simulink subsystem "State_Estimator"  (R2025b)
settings: Solver=VariableStepAuto  StartTime=0.0  StopTime=10.0  RelTol=1e-3
undefined symbols (not defined in the file or in its folder): Cbimu_meas, DiscIntNeverNeededParam, dRb0_est, dt_control, dt_data, gi, q0_est
settings Model: Creator=kjhaydon  LastModifiedBy=Liam

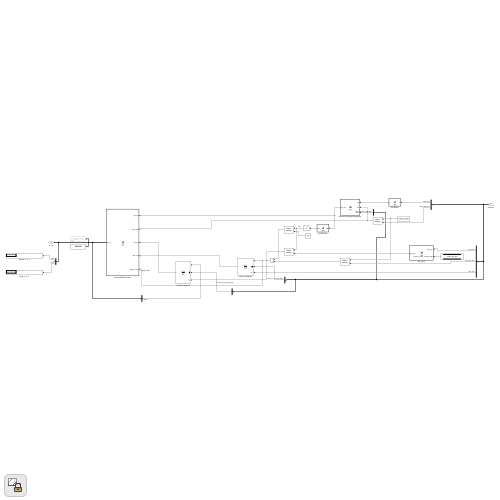
[thumbnail: Simulink's stored preview of the top-level diagram]
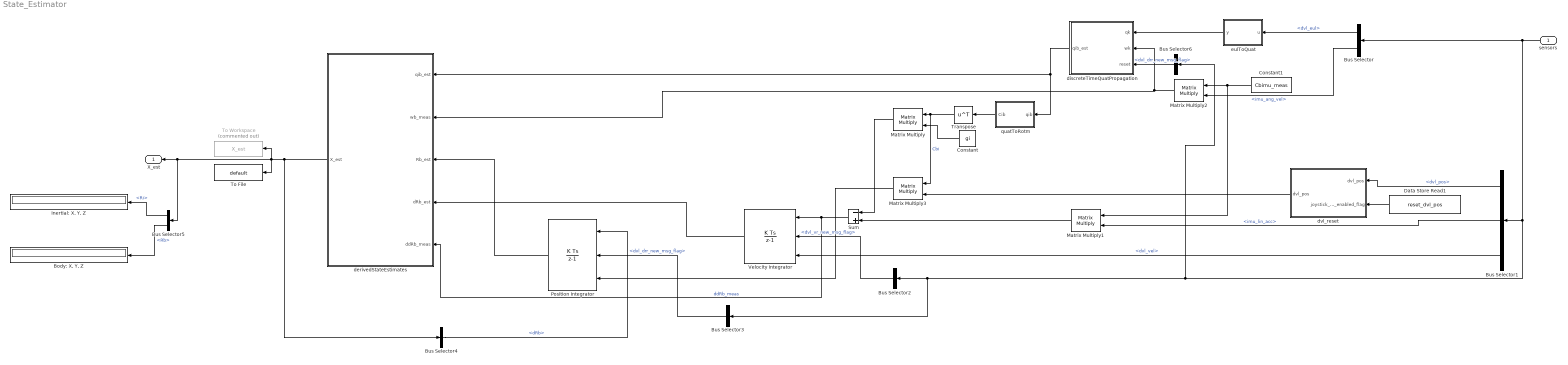
== system State_Estimator ==
  sensors : Inport  SampleTime=dt_control
  "Body: X, Y, Z" : Display
  Bus Selector : BusSelector  OutputSignals=dvl_eul,imu_ang_vel
  Bus Selector1 : BusSelector  OutputSignals=dvl_pos,imu_lin_acc,dvl_vel
  Bus Selector2 : BusSelector  OutputSignals=dvl_vr_new_msg_flag
  Bus Selector3 : BusSelector  OutputSignals=dvl_drr_new_msg_flag
  Bus Selector4 : BusSelector  OutputSignals=dRb
  Bus Selector5 : BusSelector  OutputSignals=Ri,Eul,Rb
  Bus Selector6 : BusSelector  OutputSignals=dvl_drr_new_msg_flag
  Constant : Constant  Value=gi
  Constant1 : Constant  Value=Cbimu_meas
  Data Store Read1 : DataStoreRead  DataStoreName=reset_dvl_pos  IndexOptions=Index vector (dialog)  Indices=1  OutputSizes=1
  "Inertial: X, Y, Z" : Display
  Matrix Multiply{,1..3} (4 alike) : Product  Multiplication=Matrix(*)
  Position Integrator : DiscreteIntegrator  ExternalReset=rising  InitialConditionSource=external  InitialCondition=dRb0_est  SampleTime=dt_control  ICPrevOutput=DiscIntNeverNeededParam  ICPrevScaledInput=DiscIntNeverNeededParam
  Sum : Sum  Inputs=-+
  To File : ToFile  Filename=default  MatrixName=X_est  SaveFormat=Timeseries  SampleTime=dt_data
  To Workspace : ToWorkspace  Commented=on  VariableName=X_est  SaveFormat=Timeseries  SampleTime=dt_data
  Transpose : Math  Operator=transpose
  Velocity Integrator : DiscreteIntegrator  ExternalReset=rising  InitialConditionSource=external  InitialCondition=dRb0_est  SampleTime=dt_control  ICPrevOutput=DiscIntNeverNeededParam  ICPrevScaledInput=DiscIntNeverNeededParam
  derivedStateEstimates : MATLAB Function  TreatAsAtomicUnit=on
  discreteTimeQuatPropagation : MATLAB Function  TreatAsAtomicUnit=on
  dvl_reset : MATLAB Function  TreatAsAtomicUnit=on
  eulToQuat : MATLAB Function  TreatAsAtomicUnit=on
  quatToRotm : MATLAB Function  TreatAsAtomicUnit=on
  X_est : Outport  SampleTime=dt_control
  wires:
  sensors/1 -> Bus Selector1/1, Bus Selector3/1, Bus Selector2/1, Bus Selector6/1, Bus Selector/1
  eulToQuat/1(y) -> discreteTimeQuatPropagation/1(qk)
  Velocity Integrator/1 -> derivedStateEstimates/4(dRb_est)
  discreteTimeQuatPropagation/1(qib_est) -> quatToRotm/1(qib), derivedStateEstimates/1(qib_est)
  Position Integrator/1 -> derivedStateEstimates/3(Rb_est)
  quatToRotm/1(Cib) -> Transpose/1
  Constant/1 -> Matrix Multiply/2
  Transpose/1 -> Matrix Multiply/1, Matrix Multiply3/1  "Cbi"
  Matrix Multiply/1 -> Sum/1
  Sum/1 -> Velocity Integrator/1, derivedStateEstimates/5(ddRb_meas)  "ddRb_meas"
  Bus Selector1/2 -> Matrix Multiply1/2  "<imu_lin_acc>"
  Matrix Multiply1/1 -> Sum/2
  Constant1/1 -> Matrix Multiply2/1, Matrix Multiply1/1
  Bus Selector/2 -> Matrix Multiply2/2  "<imu_ang_vel>"
  Matrix Multiply2/1 -> discreteTimeQuatPropagation/2(wk), derivedStateEstimates/2(wb_meas)
  Bus Selector1/1 -> dvl_reset/1("dvl_pos ")  "<dvl_pos>"
  Bus Selector/1 -> eulToQuat/1(u)  "<dvl_eul>"
  Bus Selector6/1 -> discreteTimeQuatPropagation/3(reset)  "<dvl_drr_new_msg_flag>"
  Bus Selector2/1 -> Velocity Integrator/2  "<dvl_vr_new_msg_flag>"
  Bus Selector3/1 -> Position Integrator/2  "<dvl_drr_new_msg_flag>"
  Bus Selector1/3 -> Velocity Integrator/3  "<dvl_vel>"
  derivedStateEstimates/1(X_est) -> X_est/1, Bus Selector5/1, To File/1, To Workspace/1, Bus Selector4/1
  Bus Selector4/1 -> Position Integrator/1  "<dRb>"
  Bus Selector5/1 -> "Inertial: X, Y, Z"/1  "<Ri>"
  Bus Selector5/3 -> "Body: X, Y, Z"/1  "<Rb>"
  dvl_reset/1(dvl_pos) -> Matrix Multiply3/2
  Matrix Multiply3/1 -> Position Integrator/3
  Data Store Read1/1 -> dvl_reset/2(joystick_mode_enabled_flag)

== matlab function State_Estimator/discreteTimeQuatPropagation ==
  settings: updateMethod=DISCRETE  sampleTime=dt_control
  data: qk input; qib_est output; wk input; reset input; q0_est parameter; dt_control parameter
function qib_est = fcn(qk, wk, reset, q0_est, dt_control)

qib_est = discreteTimeQuatPropagation(qk, wk, reset, q0_est, dt_control);

== matlab function State_Estimator/eulToQuat ==
  data: u input; y output
function y = fcn(u)

y = eulToQuat(u);

== matlab function State_Estimator/derivedStateEstimates ==
  settings: updateMethod=DISCRETE  sampleTime=dt_control
  data: qib_est input; X_est output Bus: X_bus; wb_meas input; Rb_est input; dRb_est input; ddRb_meas input
function X_est = fcn(qib_est, wb_meas, Rb_est, dRb_est, ddRb_meas)

X_est = derivedStateEstimates(qib_est, wb_meas, Rb_est, dRb_est, ddRb_meas);

== matlab function State_Estimator/quatToRotm ==
  data: qib input; Cib output
function Cib = fcn(qib)

Cib = quatToRotm(qib);

== matlab function State_Estimator/dvl_reset ==
  data: dvl_pos input; joystick_mode_enabled_flag input; dvl_pos output
function dvl_pos = fcn(dvl_pos, joystick_mode_enabled_flag)
%{
Reset the dvl position used for the state estimator.
%}
persistent offset;
persistent prior_flag;

if (isempty(offset))
    offset = [0;0;0];
end
if (isempty(prior_flag))
    prior_flag = true;
end

%switch on falling edge
if((prior_flag && ~joystick_mode_enabled_flag))
    offset = dvl_pos;
end

dvl_pos = dvl_pos - offset;
prior_flag = joystick_mode_enabled_flag;
